simulink model "PembelajaranElinHariIni"  (R2021a)
settings: Solver=VariableStepAuto  StartTime=0.0  StopTime=50  RelTol=1e-3
values from neighbouring files (symbols this model uses):
  M = 500000    [Ali.m]    (also in UmichiganLab.m = 1000; ali2.m)
settings Model: Creator=asus  LastModifiedBy=asus

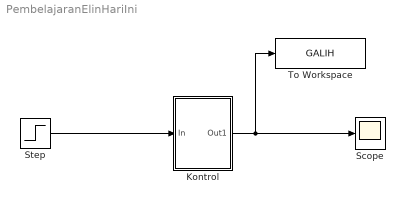
== system PembelajaranElinHariIni ==
  Kontrol : Subsystem  mask(cruish control (control system)){m=900, b=50}
      mask prompts: m "massa(kg)"; b "Redaman(N.s/m)"
      mask help: user dapat mengubah nilai dari massa dan redaman nya
      mask init:
      | m>0
      | b>0
      | m<1000
      mask Display: image("C:\Users\asus\Downloads\Ferrari.jpeg")
  Scope : Scope
  Step : Step  SampleTime=0
  To Workspace : ToWorkspace  VariableName=GALIH  SampleTime=-1
  wires:
  Step/1 -> Kontrol/1(In)
  Kontrol/1(Out1) -> To Workspace/1, Scope/1

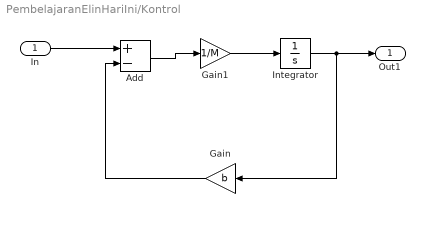
== system PembelajaranElinHariIni/Kontrol ==
  In : Inport
  Add : Sum  Inputs=+-
  Gain : Gain  Gain=b
  Gain1 : Gain  Gain=1/M
  Integrator : Integrator
  Out1 : Outport
  wires:
  Gain1/1 -> Integrator/1
  Integrator/1 -> Out1/1, Gain/1
  Gain/1 -> Add/2
  Add/1 -> Gain1/1
  In/1 -> Add/1
